simulink model "Evitar_Paredes_ACT"  (R2023b)
settings: Solver=FixedStepAuto  StartTime=0.0  StopTime=inf  RelTol=1e-3  EnableMultiTasking=on
settings Model: ExtModeTrigDuration=2  Creator=Alberto  LastModifiedBy=Alberto
settings OptimizationCC: EnhancedBackFolding=on  PassReuseOutputArgsAs=Individual arguments  ZeroExternalMemoryAtStartup=off  ZeroInternalMemoryAtStartup=off  MaxStackSize=64  OptimizeBlockOrder=speed  DifferentSizesBufferReuse=on  OptimizationCustomize=off  EfficientTunableParamExpr=on
settings DebuggingCC: ParameterOverflowMsg=none  ParameterTunabilityLossMsg=error
settings HardwareCC: ProdBitPerInt=16  ProdBitPerPointer=16  ProdBitPerSizeT=16  ProdBitPerPtrDiffT=16  ProdLargestAtomicFloat=None  ProdWordSize=8  ProdHWDeviceType=Atmel->AVR  UseEmbeddedCoderFeatures=off  UseSimulinkCoderFeatures=off
settings SFSimCC: MATLABDynamicMemAlloc=off
settings RTWCC: Description=Embedded Coder  SystemTargetFile=ert.tlc  HardwareBoard=Arduino Mega 2560  TemplateMakefile=ert_default_tmf  Toolchain=Arduino AVR  BuildConfiguration=Faster Runs
settings CodeAppCC: ForceParamTrailComments=on  IgnoreCustomStorageClasses=off  OperatorAnnotations=on  SimulinkDataObjDesc=on  SFDataObjDesc=on  MangleLength=10  InsertBlockDesc=on
settings ERTTargetCC: SupportContinuousTime=on  SupportNonInlinedSFcns=on  SupportVariableSizeSignals=on  ExtModeTransport=3  ExtModeStaticAlloc=on  ExtModeAutomaticAllocSize=off  ExtModeStaticAllocSize=2048  ExtModeMexFile=ext_xcp  ExtModeIntrfLevel=Level2 - Open

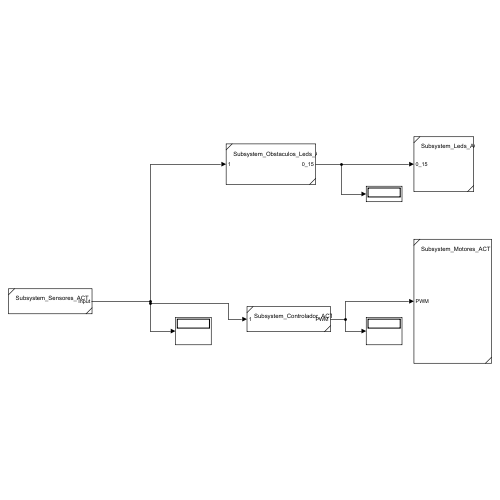
[thumbnail: Simulink's stored preview of the top-level diagram]
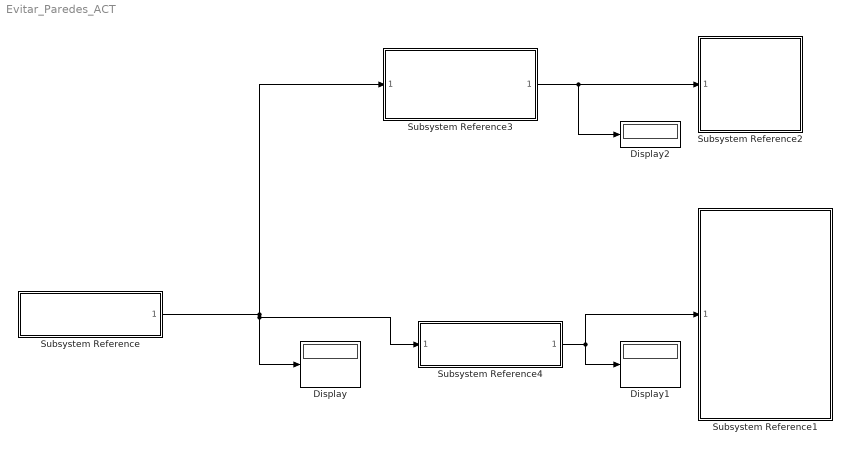
== system Evitar_Paredes_ACT ==
  Display : Display
  Display1 : Display
  Display2 : Display
  Subsystem Reference : Subsystem  ReferencedSubsystem=Subsystem_Sensores_ACT
  Subsystem Reference1 : Subsystem  ReferencedSubsystem=Subsystem_Motores_ACT
  Subsystem Reference2 : Subsystem  ReferencedSubsystem=Subsystem_Leds_ACT
  Subsystem Reference3 : Subsystem  ReferencedSubsystem=Subsystem_Obstaculos_Leds_ACT
  Subsystem Reference4 : Subsystem  ReferencedSubsystem=Subsystem_Controlador_ACT
  wires:
  Subsystem Reference/1 -> Display/1, Subsystem Reference4/1, Subsystem Reference3/1
  Subsystem Reference3/1 -> Display2/1, Subsystem Reference2/1
  Subsystem Reference4/1 -> Subsystem Reference1/1, Display1/1
